simulink model "dut_v7"  (R2023a)
settings: Solver=VariableStepAuto  StartTime=0.0  StopTime=1.0  RelTol=1e-3
undefined symbols (not defined in the file): DiscIntNeverNeededParam, Fs
libraries: hdlsllib x1, simulink_extras x1
settings Model: Creator=pj  LastModifiedBy=maarikazuki
settings ModelReferenceCC: EnableRefExpFcnMdlSchedulingChecks=on

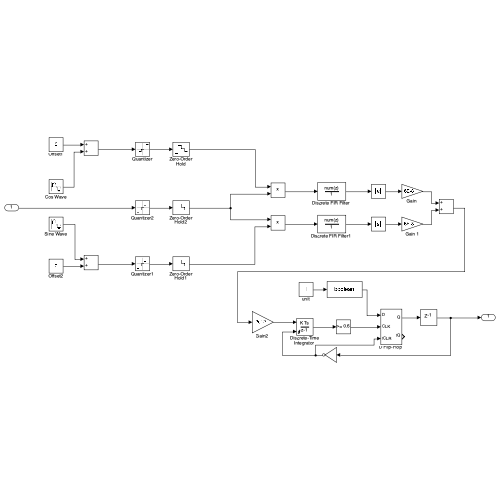
[thumbnail: Simulink's stored preview of the top-level diagram]
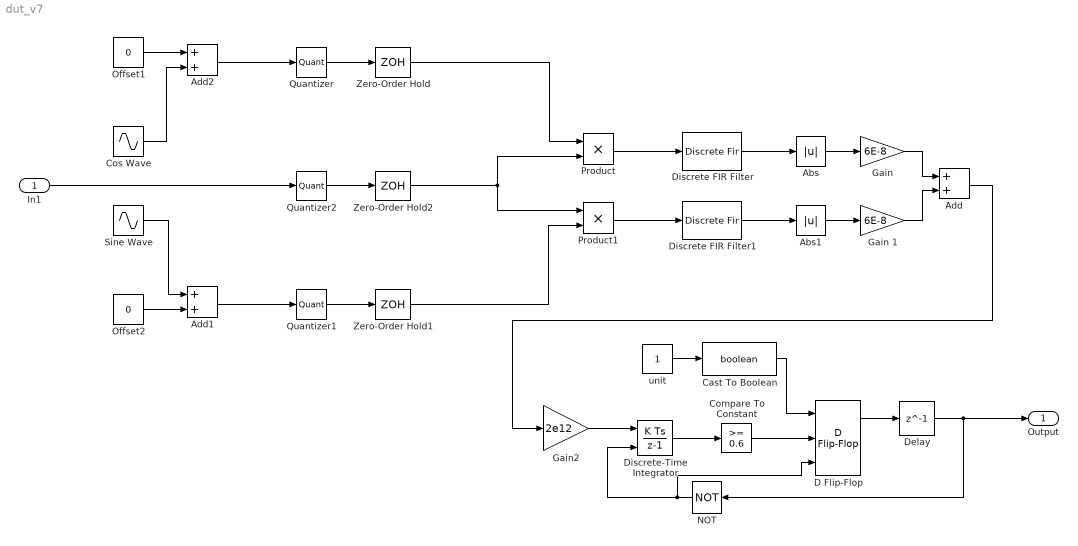
== system dut_v7 ==
  In1 : Inport
  Abs : Abs  SaturateOnIntegerOverflow=off
  Abs1 : Abs  SaturateOnIntegerOverflow=off
  Add : Sum
  Add1 : Sum
  Add2 : Sum
  Cast To Boolean : DataTypeConversion  OutDataTypeStr=boolean  SaturateOnIntegerOverflow=off  RndMeth=Floor
  Compare To Constant : hdlsllib/Logic and Bit Operations/Compare To Constant  relop=>=  const=0.6  OutDataTypeStr=boolean
  Cos Wave : Sin  Frequency=2*pi*500  Phase=pi/2  SampleTime=1/Fs
  "D Flip-Flop " : simulink_extras/Flip Flops/D Flip-Flop
  Delay : Delay  DelayLength=1
  "Discrete FIR Filter " : DiscreteFir  Coefficients="[0.00025758\t1.30E-05\t1.32E-05\t1.36E-05\t1.38E-05\t1.42E-05\t1.45E-05\t1.49E-05\t1.51E-05\t1.56E-05\t1.58E-05\t1.63E-05\t1.66E-05\t1.71E-05\t1.74E-05\t1.79E-05\t1.82E-05\t1.87E-05\t1.88E-05\t1.93E-05\t1.99E-05\t2.02E-05\t2.06E-05\t2.11E-05\t2.15E-05\t2.20E-05\t2.24E-05\t2.29E-05\t2.33E-05\t2.39E-05\t2.42E-05\t2.48E-05\t2.52E-05\t2.57E-05\t2.61E-05\t2.67E-05\t2.72E-05\t2.78E-05\t2.82E-05\t2.88E-05\t2.93E-05\t2.99E-05\t3.03E-05\t3.10E-05\t3.15E-05\t3.21E-05\t3.26E-05\t3.32E-05\t3.37E-05\t3.44E-05\t3.49E-05\t3.56E-05\t3.62E-05\t3.69E-05\t3.74E-05\t3.81E-05\t3.87E-05\t3.94E-05\t4.00E-05\t4.07E-05\t4.13E-05\t4.20E-05\t4.27E-05\t4.34E-05\t4.40E-05\t4.48E-05\t4.55E-05\t4.62E-05\t4.69E-05\t4.77E-05\t4.84E-05\t4.92E-05\t4.99E-05\t5.07E-05\t5.14E-05\t5.22E-05\t5.30E-05\t5.38E-05\t5.45E-05\t5.54E-05\t5.62E-05\t5.71E-05\t5.78E-05\t5.88E-05\t5.95E-05\t6.05E-05\t6.13E-05\t6.22E-05\t6.30E-05\t6.40E-05\t6.48E-05\t6.58E-05\t6.66E-05\t6.76E-05\t6.85E-05\t6.95E-05\t7.04E-05\t7.14E-05\t7.23E-05\t7.34E-05\t7.43E-05\t7.53E-05\t7.63E-05\t7.73E-05\t7.83E-05\t7.94E-05\t8.04E-05\t8.15E-05\t8.25E-05\t8.36E-05\t8.46E-05\t8.57E-05\t8.68E-05\t8.79E-05\t8.90E-05\t9.01E-05\t9.12E-05\t9.24E-05\t9.35E-05\t9.47E-05\t9.58E-05\t9.70E-05\t9.81E-05\t9.94E-05\t0.00010053\t0.00010181\t0.00010296\t0.00010425\t0.00010542\t0.00010673\t0.00010792\t0.00010925\t0.00011046\t0.00011181\t0.00011304\t0.0001144\t0.00011566\t0.00011704\t0.00011832\t0.00011972\t0.00012101\t0.00012243\t0.00012374\t0.00012519\t0.00012652\t0.00012798\t0.00012933\t0.00013081\t0.00013218\t0.00013368\t0.00013507\t0.00013659\t0.000138\t0.00013954\t0.00014097\t0.00014253\t0.00014398\t0.00014556\t0.00014703\t0.00014863\t0.00015012\t0.00015173\t0.00015325\t0.00015488\t0.00015642\t0.00015807\t0.00015963\t0.0001613\t0.00016288\t0.00016457\t0.00016617\t0.00016788\t0.0001695\t0.00017123\t0.00017287\t0.00017462\t0.00017628\t0.00017805\t0.00017974\t0.00018153\t0.00018323\t0.00018504\t0.00018676\t0.00018859\t0.00019034\t0.00019218\t0.00019395\t0.00019582\t0.00019761\t0.00019949\t0.0002013\t0.00020321\t0.00020504\t0.00020697\t0.00020882\t0.00021077\t0.00021264\t0.00021461\t0.0002165\t0.00021849\t0.0002204\t0.00022241\t0.00022434\t0.00022637\t0.00022832\t0.00023037\t0.00023235\t0.00023441\t0.00023641\t0.00023849\t0.00024051\t0.00024261\t0.00024465\t0.00024678\t0.00024883\t0.00025098\t0.00025306\t0.00025522\t0.00025732\t0.0002595\t0.00026162\t0.00026382\t0.00026596\t0.00026818\t0.00027034\t0.00027258\t0.00027476\t0.00027701\t0.00027921\t0.00028149\t0.00028371\t0.000286\t0.00028824\t0.00029056\t0.00029282\t0.00029515\t0.00029743\t0.00029978\t0.00030207\t0.00030444\t0.00030676\t0.00030915\t0.00031148\t0.00031389\t0.00031624\t0.00031866\t0.00032104\t0.00032348\t0.00032587\t0.00032833\t0.00033074\t0.00033322\t0.00033565\t0.00033814\t0.00034059\t0.0003431\t0.00034556\t0.00034809\t0.00035058\t0.00035312\t0.00035562\t0.00035819\t0.00036071\t0.00036328\t0.00036582\t0.00036842\t0.00037097\t0.00037358\t0.00037615\t0.00037878\t0.00038137\t0.00038401\t0.00038662\t0.00038927\t0.00039189\t0.00039457\t0.00039721\t0.0003999\t0.00040255\t0.00040525\t0.00040792\t0.00041064\t0.00041333\t0.00041606\t0.00041876\t0.00042151\t0.00042422\t0.00042699\t0.00042972\t0.00043249\t0.00043524\t0.00043803\t0.00044079\t0.00044359\t0.00044636\t0.00044918\t0.00045197\t0.0004548\t0.0004576\t0.00046044\t0.00046325\t0.00046611\t0.00046894\t0.0004718\t0.00047464\t0.00047752\t0.00048037\t0.00048327\t0.00048613\t0.00048903\t0.00049191\t0.00049482\t0.00049771\t0.00050063\t0.00050353\t0.00050647\t0.00050938\t0.00051232\t0.00051524\t0.0005182\t0.00052113\t0.0005241\t0.00052703\t0.00053001\t0.00053296\t0.00053595\t0.0005389\t0.0005419\t0.00054486\t0.00054787\t0.00055084\t0.00055386\t0.00055684\t0.00055986\t0.00056285\t0.00056588\t0.00056888\t0.00057191\t0.00057492\t0.00057796\t0.00058097\t0.00058402\t0.00058704\t0.0005901\t0.00059312\t0.00059618\t0.00059922\t0.00060228\t0.00060532\t0.00060839\t0.00061144\t0.00061451\t0.00061756\t0.00062064\t0.00062369\t0.00062678\t0.00062984\t0.00063293\t0.00063599\t0.00063908\t0.00064214\t0.00064524\t0.00064831\t0.0006514\t0.00065447\t0.00065757\t0.00066065\t0.00066375\t0.00066682\t0.00066993\t0.000673\t0.00067611\t0.00067919\t0.00068229\t0.00068537\t0.00068847\t0.00069155\t0.00069466\t0.00069774\t0.00070084\t0.00070392\t0.00070702\t0.0007101\t0.0007132\t0.00071628\t0.00071938\t0.00072245\t0.00072555\t0.00072862\t0.00073172\t0.00073479\t0.00073788\t0.00074094\t0.00074404\t0.0007471\t0.00075018\t0.00075324\t0.00075632\t0.00075938\t0.00076246\t0.0007655\t0.00076858\t0.00077162\t0.00077469\t0.00077773\t0.00078079\t0.00078382\t0.00078688\t0.0007899\t0.00079295\t0.00079597\t0.00079902\t0.00080203\t0.00080506\t0.00080807\t0.00081109\t0.00081409\t0.00081711\t0.00082009\t0.00082311\t0.00082608\t0.00082909\t0.00083205\t0.00083505\t0.000838\t0.00084099\t0.00084394\t0.00084691\t0.00084985\t0.00085281\t0.00085573\t0.00085868\t0.0008616\t0.00086454\t0.00086744\t0.00087037\t0.00087326\t0.00087617\t0.00087905\t0.00088195\t0.00088481\t0.0008877\t0.00089055\t0.00089342\t0.00089626\t0.00089912\t0.00090194\t0.00090479\t0.00090759\t0.00091042\t0.00091321\t0.00091603\t0.0009188\t0.0009216\t0.00092436\t0.00092714\t0.00092989\t0.00093265\t0.00093538\t0.00093812\t0.00094083\t0.00094356\t0.00094625\t0.00094896\t0.00095164\t0.00095433\t0.00095698\t0.00095966\t0.00096229\t0.00096495\t0.00096756\t0.0009702\t0.00097279\t0.0009754\t0.00097798\t0.00098057\t0.00098313\t0.0009857\t0.00098823\t0.00099079\t0.0009933\t0.00099583\t0.00099832\t0.0010008\t0.0010033\t0.0010058\t0.0010082\t0.0010107\t0.0010131\t0.0010155\t0.0010179\t0.0010204\t0.0010227\t0.0010251\t0.0010275\t0.0010298\t0.0010322\t0.0010345\t0.0010368\t0.0010391\t0.0010414\t0.0010437\t0.0010459\t0.0010482\t0.0010504\t0.0010527\t0.0010549\t0.0010571\t0.0010592\t0.0010614\t0.0010636\t0.0010657\t0.0010678\t0.00107\t0.0010721\t0.0010742\t0.0010762\t0.0010783\t0.0010803\t0.0010824\t0.0010844\t0.0010864\t0.0010883\t0.0010903\t0.0010923\t0.0010942\t0.0010961\t0.0010981\t0.0011\t0.0011018\t0.0011037\t0.0011056\t0.0011074\t0.0011092\t0.001111\t0.0011128\t0.0011146\t0.0011163\t0.0011181\t0.0011198\t0.0011215\t0.0011232\t0.0011249\t0.0011265\t0.0011282\t0.0011298\t0.0011314\t0.001133\t0.0011346\t0.0011362\t0.0011377\t0.0011392\t0.0011407\t0.0011422\t0.0011437\t0.0011452\t0.0011466\t0.001148\t0.0011494\t0.0011508\t0.0011522\t0.0011536\t0.0011549\t0.0011562\t0.0011575\t0.0011588\t0.0011601\t0.0011613\t0.0011626\t0.0011638\t0.001165\t0.0011662\t0.0011673\t0.0011685\t0.0011696\t0.0011707\t0.0011718\t0.0011729\t0.0011739\t0.0011749\t0.0011759\t0.0011769\t0.0011779\t0.0011789\t0.0011798\t0.0011808\t0.0011816\t0.0011825\t0.0011834\t0.0011843\t0.0011851\t0.0011859\t0.0011867\t0.0011875\t0.0011882\t0.0011889\t0.0011897\t0.0011904\t0.001191\t0.0011917\t0.0011923\t0.001193\t0.0011936\t0.0011941\t0.0011947\t0.0011953\t0.0011958\t0.0011963\t0.0011968\t0.0011972\t0.0011977\t0.0011981\t0.0011985\t0.0011989\t0.0011993\t0.0011996\t0.0012\t0.0012003\t0.0012006\t0.0012008\t0.0012011\t0.0012013\t0.0012015\t0.0012017\t0.0012019\t0.0012021\t0.0012022\t0.0012023\t0.0012024\t0.0012025\t0.0012026\t0.0012026\t0.0012026\t0.0012026\t0.0012026\t0.0012026\t0.0012025\t0.0012024\t0.0012023\t0.0012022\t0.0012021\t0.0012019\t0.0012017\t0.0012015\t0.0012013\t0.0012011\t0.0012008\t0.0012006\t0.0012003\t0.0012\t0.0011996\t0.0011993\t0.0011989\t0.0011985\t0.0011981\t0.0011977\t0.0011972\t0.0011968\t0.0011963\t0.0011958\t0.0011953\t0.0011947\t0.0011941\t0.0011936\t0.001193\t0.0011923\t0.0011917\t0.001191\t0.0011904\t0.0011897\t0.0011889\t0.0011882\t0.0011875\t0.0011867\t0.0011859\t0.0011851\t0.0011843\t0.0011834\t0.0011825\t0.0011816\t0.0011808\t0.0011798\t0.0011789\t0.0011779\t0.0011769\t0.0011759\t0.0011749\t0.0011739\t0.0011729\t0.0011718\t0.0011707\t0.0011696\t0.0011685\t0.0011673\t0.0011662\t0.001165\t0.0011638\t0.0011626\t0.0011613\t0.0011601\t0.0011588\t0.0011575\t0.0011562\t0.0011549\t0.0011536\t0.0011522\t0.0011508\t0.0011494\t0.001148\t0.0011466\t0.0011452\t0.0011437\t0.0011422\t0.0011407\t0.0011392\t0.0011377\t0.0011362\t0.0011346\t0.001133\t0.0011314\t0.0011298\t0.0011282\t0.0011265\t0.0011249\t0.0011232\t0.0011215\t0.0011198\t0.0011181\t0.0011163\t0.0011146\t0.0011128\t0.001111\t0.0011092\t0.0011074\t0.0011056\t0.0011037\t0.0011018\t0.0011\t0.0010981\t0.0010961\t0.0010942\t0.0010923\t0.0010903\t0.0010883\t0.0010864\t0.0010844\t0.0010824\t0.0010803\t0.0010783\t0.0010762\t0.0010742\t0.0010721\t0.00107\t0.0010678\t0.0010657\t0.0010636\t0.0010614\t0.0010592\t0.0010571\t0.0010549\t0.0010527\t0.0010504\t0.0010482\t0.0010459\t0.0010437\t0.0010414\t0.0010391\t0.0010368\t0.0010345\t0.0010322\t0.0010298\t0.0010275\t0.0010251\t0.0010227\t0.0010204\t0.0010179\t0.0010155\t0.0010131\t0.0010107\t0.0010082\t0.0010058\t0.0010033\t0.0010008\t0.00099832\t0.00099583\t0.0009933\t0.00099079\t0.00098823\t0.0009857\t0.00098313\t0.00098057\t0.00097798\t0.0009754\t0.00097279\t0.0009702\t0.00096756\t0.00096495\t0.00096229\t0.00095966\t0.00095698\t0.00095433\t0.00095164\t0.00094896\t0.00094625\t0.00094356\t0.00094083\t0.00093812\t0.00093538\t0.00093265\t0.00092989\t0.00092714\t0.00092436\t0.0009216\t0.0009188\t0.00091603\t0.00091321\t0.00091042\t0.00090759\t0.00090479\t0.00090194\t0.00089912\t0.00089626\t0.00089342\t0.00089055\t0.0008877\t0.00088481\t0.00088195\t0.00087905\t0.00087617\t0.00087326\t0.00087037\t0.00086744\t0.00086454\t0.0008616\t0.00085868\t0.00085573\t0.00085281\t0.00084985\t0.00084691\t0.00084394\t0.00084099\t0.000838\t0.00083505\t0.00083205\t0.00082909\t0.00082608\t0.00082311\t0.00082009\t0.00081711\t0.00081409\t0.00081109\t0.00080807\t0.00080506\t0.00080203\t0.00079902\t0.00079597\t0.00079295\t0.0007899\t0.00078688\t0.00078382\t0.00078079\t0.00077773\t0.00077469\t0.00077162\t0.00076858\t0.0007655\t0.00076246\t0.00075938\t0.00075632\t0.00075324\t0.00075018\t0.0007471\t0.00074404\t0.00074094\t0.00073788\t0.00073479\t0.00073172\t0.00072862\t0.00072555\t0.00072245\t0.00071938\t0.00071628\t0.0007132\t0.0007101\t0.00070702\t0.00070392\t0.00070084\t0.00069774\t0.00069466\t0.00069155\t0.00068847\t0.00068537\t0.00068229\t0.00067919\t0.00067611\t0.000673\t0.00066993\t0.00066682\t0.00066375\t0.00066065\t0.00065757\t0.00065447\t0.0006514\t0.00064831\t0.00064524\t0.00064214\t0.00063908\t0.00063599\t0.00063293\t0.00062984\t0.00062678\t0.00062369\t0.00062064\t0.00061756\t0.00061451\t0.00061144\t0.00060839\t0.00060532\t0.00060228\t0.00059922\t0.00059618\t0.00059312\t0.0005901\t0.00058704\t0.00058402\t0.00058097\t0.00057796\t0.00057492\t0.00057191\t0.00056888\t0.00056588\t0.00056285\t0.00055986\t0.00055684\t0.00055386\t0.00055084\t0.00054787\t0.00054486\t0.0005419\t0.0005389\t0.00053595\t0.00053296\t0.00053001\t0.00052703\t0.0005241\t0.00052113\t0.0005182\t0.00051524\t0.00051232\t0.00050938\t0.00050647\t0.00050353\t0.00050063\t0.00049771\t0.00049482\t0.00049191\t0.00048903\t0.00048613\t0.00048327\t0.00048037\t0.00047752\t0.00047464\t0.0004718\t0.00046894\t0.00046611\t0.00046325\t0.00046044\t0.0004576\t0.0004548\t0.00045197\t0.00044918\t0.00044636\t0.00044359\t0.00044079\t0.00043803\t0.00043524\t0.00043249\t0.00042972\t0.00042699\t0.00042422\t0.00042151\t0.00041876\t0.00041606\t0.00041333\t0.00041064\t0.00040792\t0.00040525\t0.00040255\t0.0003999\t0.00039721\t0.00039457\t0.00039189\t0.00038927\t0.00038662\t0.00038401\t0.00038137\t0.00037878\t0.00037615\t0.00037358\t0.00037097\t0.00036842\t0.00036582\t0.00036328\t0.00036071\t0.00035819\t0.00035562\t0.00035312\t0.00035058\t0.00034809\t0.00034556\t0.0003431\t0.00034059\t0.00033814\t0.00033565\t0.00033322\t0.00033074\t0.00032833\t0.00032587\t0.00032348\t0.00032104\t0.00031866\t0.00031624\t0.00031389\t0.00031148\t0.00030915\t0.00030676\t0.00030444\t0.00030207\t0.00029978\t0.00029743\t0.00029515\t0.00029282\t0.00029056\t0.00028824\t0.000286\t0.00028371\t0.00028149\t0.00027921\t0.00027701\t0.00027476\t0.00027258\t0.00027034\t0.00026818\t0.00026596\t0.00026382\t0.00026162\t0.0002595\t0.00025732\t0.00025522\t0.00025306\t0.00025098\t0.00024883\t0.00024678\t0.00024465\t0.00024261\t0.00024051\t0.00023849\t0.00023641\t0.00023441\t0.00023235\t0.00023037\t0.00022832\t0.00022637\t0.00022434\t0.00022241\t0.0002204\t0.00021849\t0.0002165\t0.00021461\t0.00021264\t0.00021077\t0.00020882\t0.00020697\t0.00020504\t0.00020321\t0.0002013\t0.00019949\t0.00019761\t0.00019582\t0.00019395\t0.00019218\t0.00019034\t0.00018859\t0.00018676\t0.00018504\t0.00018323\t0.00018153\t0.00017974\t0.00017805\t0.00017628\t0.00017462\t0.00017287\t0.00017123\t0.0001695\t0.00016788\t0.00016617\t0.00016457\t0.00016288\t0.0001613\t0.00015963\t0.00015807\t0.00015642\t0.00015488\t0.00015325\t0.00015173\t0.00015012\t0.00014863\t0.00014703\t0.00014556\t0.00014398\t0.00014253\t0.00014097\t0.00013954\t0.000138\t0.00013659\t0.00013507\t0.00013368\t0.00013218\t0.00013081\t0.00012933\t0.00012798\t0.00012652\t0.00012519\t0.00012374\t0.00012243\t0.00012101\t0.00011972\t0.00011832\t0.00011704\t0.00011566\t0.0001144\t0.00011304\t0.00011181\t0.00011046\t0.00010925\t0.00010792\t0.00010673\t0.00010542\t0.00010425\t0.00010296\t0.00010181\t0.00010053\t9.94E-05\t9.81E-05\t9.70E-05\t9.58E-05\t9.47E-05\t9.35E-05\t9.24E-05\t9.12E-05\t9.01E-05\t8.90E-05\t8.79E-05\t8.68E-05\t8.57E-05\t8.46E-05\t8.36E-05\t8.25E-05\t8.15E-05\t8.04E-05\t7.94E-05\t7.83E-05\t7.73E-05\t7.63E-05\t7.53E-05\t7.43E-05\t7.34E-05\t7.23E-05\t7.14E-05\t7.04E-05\t6.95E-05\t6.85E-05\t6.76E-05\t6.66E-05\t6.58E-05\t6.48E-05\t6.40E-05\t6.30E-05\t6.22E-05\t6.13E-05\t6.05E-05\t5.95E-05\t5.88E-05\t5.78E-05\t5.71E-05\t5.62E-05\t5.54E-05\t5.45E-05\t5.38E-05\t5.30E-05\t5.22E-05\t5.14E-05\t5.07E-05\t4.99E-05\t4.92E-05\t4.84E-05\t4.77E-05\t4.69E-05\t4.62E-05\t4.55E-05\t4.48E-05\t4.40E-05\t4.34E-05\t4.27E-05\t4.20E-05\t4.13E-05\t4.07E-05\t4.00E-05\t3.94E-05\t3.87E-05\t3.81E-05\t3.74E-05\t3.69E-05\t3.62E-05\t3.56E-05\t3.49E-05\t3.44E-05\t3.37E-05\t3.32E-05\t3.26E-05\t3.21E-05\t3.15E-05\t3.10E-05\t3.03E-05\t2.99E-05\t2.93E-05\t2.88E-05\t2.82E-05\t2.78E-05\t2.72E-05\t2.67E-05\t2.61E-05\t2.57E-05\t2.52E-05\t2.48E-05\t2.42E-05\t2.39E-05\t2.33E-05\t2.29E-05\t2.24E-05\t2.20E-05\t2.15E-05\t2.11E-05\t2.06E-05\t2.02E-05\t1.99E-05\t1.93E-05\t1.88E-05\t1.87E-05\t1.82E-05\t1.79E-05\t1.74E-05\t1.71E-05\t1.66E-05\t1.63E-05\t1.58E-05\t1.56E-05\t1.51E-05\t1.49E-05\t1.45E-05\t1.42E-05\t1.38E-05\t1.36E-05\t1.32E-05\t1.30E-05\t0.00025758]"
  "Discrete FIR Filter1 " : DiscreteFir  Coefficients="[0.00025758\t1.30E-05\t1.32E-05\t1.36E-05\t1.38E-05\t1.42E-05\t1.45E-05\t1.49E-05\t1.51E-05\t1.56E-05\t1.58E-05\t1.63E-05\t1.66E-05\t1.71E-05\t1.74E-05\t1.79E-05\t1.82E-05\t1.87E-05\t1.88E-05\t1.93E-05\t1.99E-05\t2.02E-05\t2.06E-05\t2.11E-05\t2.15E-05\t2.20E-05\t2.24E-05\t2.29E-05\t2.33E-05\t2.39E-05\t2.42E-05\t2.48E-05\t2.52E-05\t2.57E-05\t2.61E-05\t2.67E-05\t2.72E-05\t2.78E-05\t2.82E-05\t2.88E-05\t2.93E-05\t2.99E-05\t3.03E-05\t3.10E-05\t3.15E-05\t3.21E-05\t3.26E-05\t3.32E-05\t3.37E-05\t3.44E-05\t3.49E-05\t3.56E-05\t3.62E-05\t3.69E-05\t3.74E-05\t3.81E-05\t3.87E-05\t3.94E-05\t4.00E-05\t4.07E-05\t4.13E-05\t4.20E-05\t4.27E-05\t4.34E-05\t4.40E-05\t4.48E-05\t4.55E-05\t4.62E-05\t4.69E-05\t4.77E-05\t4.84E-05\t4.92E-05\t4.99E-05\t5.07E-05\t5.14E-05\t5.22E-05\t5.30E-05\t5.38E-05\t5.45E-05\t5.54E-05\t5.62E-05\t5.71E-05\t5.78E-05\t5.88E-05\t5.95E-05\t6.05E-05\t6.13E-05\t6.22E-05\t6.30E-05\t6.40E-05\t6.48E-05\t6.58E-05\t6.66E-05\t6.76E-05\t6.85E-05\t6.95E-05\t7.04E-05\t7.14E-05\t7.23E-05\t7.34E-05\t7.43E-05\t7.53E-05\t7.63E-05\t7.73E-05\t7.83E-05\t7.94E-05\t8.04E-05\t8.15E-05\t8.25E-05\t8.36E-05\t8.46E-05\t8.57E-05\t8.68E-05\t8.79E-05\t8.90E-05\t9.01E-05\t9.12E-05\t9.24E-05\t9.35E-05\t9.47E-05\t9.58E-05\t9.70E-05\t9.81E-05\t9.94E-05\t0.00010053\t0.00010181\t0.00010296\t0.00010425\t0.00010542\t0.00010673\t0.00010792\t0.00010925\t0.00011046\t0.00011181\t0.00011304\t0.0001144\t0.00011566\t0.00011704\t0.00011832\t0.00011972\t0.00012101\t0.00012243\t0.00012374\t0.00012519\t0.00012652\t0.00012798\t0.00012933\t0.00013081\t0.00013218\t0.00013368\t0.00013507\t0.00013659\t0.000138\t0.00013954\t0.00014097\t0.00014253\t0.00014398\t0.00014556\t0.00014703\t0.00014863\t0.00015012\t0.00015173\t0.00015325\t0.00015488\t0.00015642\t0.00015807\t0.00015963\t0.0001613\t0.00016288\t0.00016457\t0.00016617\t0.00016788\t0.0001695\t0.00017123\t0.00017287\t0.00017462\t0.00017628\t0.00017805\t0.00017974\t0.00018153\t0.00018323\t0.00018504\t0.00018676\t0.00018859\t0.00019034\t0.00019218\t0.00019395\t0.00019582\t0.00019761\t0.00019949\t0.0002013\t0.00020321\t0.00020504\t0.00020697\t0.00020882\t0.00021077\t0.00021264\t0.00021461\t0.0002165\t0.00021849\t0.0002204\t0.00022241\t0.00022434\t0.00022637\t0.00022832\t0.00023037\t0.00023235\t0.00023441\t0.00023641\t0.00023849\t0.00024051\t0.00024261\t0.00024465\t0.00024678\t0.00024883\t0.00025098\t0.00025306\t0.00025522\t0.00025732\t0.0002595\t0.00026162\t0.00026382\t0.00026596\t0.00026818\t0.00027034\t0.00027258\t0.00027476\t0.00027701\t0.00027921\t0.00028149\t0.00028371\t0.000286\t0.00028824\t0.00029056\t0.00029282\t0.00029515\t0.00029743\t0.00029978\t0.00030207\t0.00030444\t0.00030676\t0.00030915\t0.00031148\t0.00031389\t0.00031624\t0.00031866\t0.00032104\t0.00032348\t0.00032587\t0.00032833\t0.00033074\t0.00033322\t0.00033565\t0.00033814\t0.00034059\t0.0003431\t0.00034556\t0.00034809\t0.00035058\t0.00035312\t0.00035562\t0.00035819\t0.00036071\t0.00036328\t0.00036582\t0.00036842\t0.00037097\t0.00037358\t0.00037615\t0.00037878\t0.00038137\t0.00038401\t0.00038662\t0.00038927\t0.00039189\t0.00039457\t0.00039721\t0.0003999\t0.00040255\t0.00040525\t0.00040792\t0.00041064\t0.00041333\t0.00041606\t0.00041876\t0.00042151\t0.00042422\t0.00042699\t0.00042972\t0.00043249\t0.00043524\t0.00043803\t0.00044079\t0.00044359\t0.00044636\t0.00044918\t0.00045197\t0.0004548\t0.0004576\t0.00046044\t0.00046325\t0.00046611\t0.00046894\t0.0004718\t0.00047464\t0.00047752\t0.00048037\t0.00048327\t0.00048613\t0.00048903\t0.00049191\t0.00049482\t0.00049771\t0.00050063\t0.00050353\t0.00050647\t0.00050938\t0.00051232\t0.00051524\t0.0005182\t0.00052113\t0.0005241\t0.00052703\t0.00053001\t0.00053296\t0.00053595\t0.0005389\t0.0005419\t0.00054486\t0.00054787\t0.00055084\t0.00055386\t0.00055684\t0.00055986\t0.00056285\t0.00056588\t0.00056888\t0.00057191\t0.00057492\t0.00057796\t0.00058097\t0.00058402\t0.00058704\t0.0005901\t0.00059312\t0.00059618\t0.00059922\t0.00060228\t0.00060532\t0.00060839\t0.00061144\t0.00061451\t0.00061756\t0.00062064\t0.00062369\t0.00062678\t0.00062984\t0.00063293\t0.00063599\t0.00063908\t0.00064214\t0.00064524\t0.00064831\t0.0006514\t0.00065447\t0.00065757\t0.00066065\t0.00066375\t0.00066682\t0.00066993\t0.000673\t0.00067611\t0.00067919\t0.00068229\t0.00068537\t0.00068847\t0.00069155\t0.00069466\t0.00069774\t0.00070084\t0.00070392\t0.00070702\t0.0007101\t0.0007132\t0.00071628\t0.00071938\t0.00072245\t0.00072555\t0.00072862\t0.00073172\t0.00073479\t0.00073788\t0.00074094\t0.00074404\t0.0007471\t0.00075018\t0.00075324\t0.00075632\t0.00075938\t0.00076246\t0.0007655\t0.00076858\t0.00077162\t0.00077469\t0.00077773\t0.00078079\t0.00078382\t0.00078688\t0.0007899\t0.00079295\t0.00079597\t0.00079902\t0.00080203\t0.00080506\t0.00080807\t0.00081109\t0.00081409\t0.00081711\t0.00082009\t0.00082311\t0.00082608\t0.00082909\t0.00083205\t0.00083505\t0.000838\t0.00084099\t0.00084394\t0.00084691\t0.00084985\t0.00085281\t0.00085573\t0.00085868\t0.0008616\t0.00086454\t0.00086744\t0.00087037\t0.00087326\t0.00087617\t0.00087905\t0.00088195\t0.00088481\t0.0008877\t0.00089055\t0.00089342\t0.00089626\t0.00089912\t0.00090194\t0.00090479\t0.00090759\t0.00091042\t0.00091321\t0.00091603\t0.0009188\t0.0009216\t0.00092436\t0.00092714\t0.00092989\t0.00093265\t0.00093538\t0.00093812\t0.00094083\t0.00094356\t0.00094625\t0.00094896\t0.00095164\t0.00095433\t0.00095698\t0.00095966\t0.00096229\t0.00096495\t0.00096756\t0.0009702\t0.00097279\t0.0009754\t0.00097798\t0.00098057\t0.00098313\t0.0009857\t0.00098823\t0.00099079\t0.0009933\t0.00099583\t0.00099832\t0.0010008\t0.0010033\t0.0010058\t0.0010082\t0.0010107\t0.0010131\t0.0010155\t0.0010179\t0.0010204\t0.0010227\t0.0010251\t0.0010275\t0.0010298\t0.0010322\t0.0010345\t0.0010368\t0.0010391\t0.0010414\t0.0010437\t0.0010459\t0.0010482\t0.0010504\t0.0010527\t0.0010549\t0.0010571\t0.0010592\t0.0010614\t0.0010636\t0.0010657\t0.0010678\t0.00107\t0.0010721\t0.0010742\t0.0010762\t0.0010783\t0.0010803\t0.0010824\t0.0010844\t0.0010864\t0.0010883\t0.0010903\t0.0010923\t0.0010942\t0.0010961\t0.0010981\t0.0011\t0.0011018\t0.0011037\t0.0011056\t0.0011074\t0.0011092\t0.001111\t0.0011128\t0.0011146\t0.0011163\t0.0011181\t0.0011198\t0.0011215\t0.0011232\t0.0011249\t0.0011265\t0.0011282\t0.0011298\t0.0011314\t0.001133\t0.0011346\t0.0011362\t0.0011377\t0.0011392\t0.0011407\t0.0011422\t0.0011437\t0.0011452\t0.0011466\t0.001148\t0.0011494\t0.0011508\t0.0011522\t0.0011536\t0.0011549\t0.0011562\t0.0011575\t0.0011588\t0.0011601\t0.0011613\t0.0011626\t0.0011638\t0.001165\t0.0011662\t0.0011673\t0.0011685\t0.0011696\t0.0011707\t0.0011718\t0.0011729\t0.0011739\t0.0011749\t0.0011759\t0.0011769\t0.0011779\t0.0011789\t0.0011798\t0.0011808\t0.0011816\t0.0011825\t0.0011834\t0.0011843\t0.0011851\t0.0011859\t0.0011867\t0.0011875\t0.0011882\t0.0011889\t0.0011897\t0.0011904\t0.001191\t0.0011917\t0.0011923\t0.001193\t0.0011936\t0.0011941\t0.0011947\t0.0011953\t0.0011958\t0.0011963\t0.0011968\t0.0011972\t0.0011977\t0.0011981\t0.0011985\t0.0011989\t0.0011993\t0.0011996\t0.0012\t0.0012003\t0.0012006\t0.0012008\t0.0012011\t0.0012013\t0.0012015\t0.0012017\t0.0012019\t0.0012021\t0.0012022\t0.0012023\t0.0012024\t0.0012025\t0.0012026\t0.0012026\t0.0012026\t0.0012026\t0.0012026\t0.0012026\t0.0012025\t0.0012024\t0.0012023\t0.0012022\t0.0012021\t0.0012019\t0.0012017\t0.0012015\t0.0012013\t0.0012011\t0.0012008\t0.0012006\t0.0012003\t0.0012\t0.0011996\t0.0011993\t0.0011989\t0.0011985\t0.0011981\t0.0011977\t0.0011972\t0.0011968\t0.0011963\t0.0011958\t0.0011953\t0.0011947\t0.0011941\t0.0011936\t0.001193\t0.0011923\t0.0011917\t0.001191\t0.0011904\t0.0011897\t0.0011889\t0.0011882\t0.0011875\t0.0011867\t0.0011859\t0.0011851\t0.0011843\t0.0011834\t0.0011825\t0.0011816\t0.0011808\t0.0011798\t0.0011789\t0.0011779\t0.0011769\t0.0011759\t0.0011749\t0.0011739\t0.0011729\t0.0011718\t0.0011707\t0.0011696\t0.0011685\t0.0011673\t0.0011662\t0.001165\t0.0011638\t0.0011626\t0.0011613\t0.0011601\t0.0011588\t0.0011575\t0.0011562\t0.0011549\t0.0011536\t0.0011522\t0.0011508\t0.0011494\t0.001148\t0.0011466\t0.0011452\t0.0011437\t0.0011422\t0.0011407\t0.0011392\t0.0011377\t0.0011362\t0.0011346\t0.001133\t0.0011314\t0.0011298\t0.0011282\t0.0011265\t0.0011249\t0.0011232\t0.0011215\t0.0011198\t0.0011181\t0.0011163\t0.0011146\t0.0011128\t0.001111\t0.0011092\t0.0011074\t0.0011056\t0.0011037\t0.0011018\t0.0011\t0.0010981\t0.0010961\t0.0010942\t0.0010923\t0.0010903\t0.0010883\t0.0010864\t0.0010844\t0.0010824\t0.0010803\t0.0010783\t0.0010762\t0.0010742\t0.0010721\t0.00107\t0.0010678\t0.0010657\t0.0010636\t0.0010614\t0.0010592\t0.0010571\t0.0010549\t0.0010527\t0.0010504\t0.0010482\t0.0010459\t0.0010437\t0.0010414\t0.0010391\t0.0010368\t0.0010345\t0.0010322\t0.0010298\t0.0010275\t0.0010251\t0.0010227\t0.0010204\t0.0010179\t0.0010155\t0.0010131\t0.0010107\t0.0010082\t0.0010058\t0.0010033\t0.0010008\t0.00099832\t0.00099583\t0.0009933\t0.00099079\t0.00098823\t0.0009857\t0.00098313\t0.00098057\t0.00097798\t0.0009754\t0.00097279\t0.0009702\t0.00096756\t0.00096495\t0.00096229\t0.00095966\t0.00095698\t0.00095433\t0.00095164\t0.00094896\t0.00094625\t0.00094356\t0.00094083\t0.00093812\t0.00093538\t0.00093265\t0.00092989\t0.00092714\t0.00092436\t0.0009216\t0.0009188\t0.00091603\t0.00091321\t0.00091042\t0.00090759\t0.00090479\t0.00090194\t0.00089912\t0.00089626\t0.00089342\t0.00089055\t0.0008877\t0.00088481\t0.00088195\t0.00087905\t0.00087617\t0.00087326\t0.00087037\t0.00086744\t0.00086454\t0.0008616\t0.00085868\t0.00085573\t0.00085281\t0.00084985\t0.00084691\t0.00084394\t0.00084099\t0.000838\t0.00083505\t0.00083205\t0.00082909\t0.00082608\t0.00082311\t0.00082009\t0.00081711\t0.00081409\t0.00081109\t0.00080807\t0.00080506\t0.00080203\t0.00079902\t0.00079597\t0.00079295\t0.0007899\t0.00078688\t0.00078382\t0.00078079\t0.00077773\t0.00077469\t0.00077162\t0.00076858\t0.0007655\t0.00076246\t0.00075938\t0.00075632\t0.00075324\t0.00075018\t0.0007471\t0.00074404\t0.00074094\t0.00073788\t0.00073479\t0.00073172\t0.00072862\t0.00072555\t0.00072245\t0.00071938\t0.00071628\t0.0007132\t0.0007101\t0.00070702\t0.00070392\t0.00070084\t0.00069774\t0.00069466\t0.00069155\t0.00068847\t0.00068537\t0.00068229\t0.00067919\t0.00067611\t0.000673\t0.00066993\t0.00066682\t0.00066375\t0.00066065\t0.00065757\t0.00065447\t0.0006514\t0.00064831\t0.00064524\t0.00064214\t0.00063908\t0.00063599\t0.00063293\t0.00062984\t0.00062678\t0.00062369\t0.00062064\t0.00061756\t0.00061451\t0.00061144\t0.00060839\t0.00060532\t0.00060228\t0.00059922\t0.00059618\t0.00059312\t0.0005901\t0.00058704\t0.00058402\t0.00058097\t0.00057796\t0.00057492\t0.00057191\t0.00056888\t0.00056588\t0.00056285\t0.00055986\t0.00055684\t0.00055386\t0.00055084\t0.00054787\t0.00054486\t0.0005419\t0.0005389\t0.00053595\t0.00053296\t0.00053001\t0.00052703\t0.0005241\t0.00052113\t0.0005182\t0.00051524\t0.00051232\t0.00050938\t0.00050647\t0.00050353\t0.00050063\t0.00049771\t0.00049482\t0.00049191\t0.00048903\t0.00048613\t0.00048327\t0.00048037\t0.00047752\t0.00047464\t0.0004718\t0.00046894\t0.00046611\t0.00046325\t0.00046044\t0.0004576\t0.0004548\t0.00045197\t0.00044918\t0.00044636\t0.00044359\t0.00044079\t0.00043803\t0.00043524\t0.00043249\t0.00042972\t0.00042699\t0.00042422\t0.00042151\t0.00041876\t0.00041606\t0.00041333\t0.00041064\t0.00040792\t0.00040525\t0.00040255\t0.0003999\t0.00039721\t0.00039457\t0.00039189\t0.00038927\t0.00038662\t0.00038401\t0.00038137\t0.00037878\t0.00037615\t0.00037358\t0.00037097\t0.00036842\t0.00036582\t0.00036328\t0.00036071\t0.00035819\t0.00035562\t0.00035312\t0.00035058\t0.00034809\t0.00034556\t0.0003431\t0.00034059\t0.00033814\t0.00033565\t0.00033322\t0.00033074\t0.00032833\t0.00032587\t0.00032348\t0.00032104\t0.00031866\t0.00031624\t0.00031389\t0.00031148\t0.00030915\t0.00030676\t0.00030444\t0.00030207\t0.00029978\t0.00029743\t0.00029515\t0.00029282\t0.00029056\t0.00028824\t0.000286\t0.00028371\t0.00028149\t0.00027921\t0.00027701\t0.00027476\t0.00027258\t0.00027034\t0.00026818\t0.00026596\t0.00026382\t0.00026162\t0.0002595\t0.00025732\t0.00025522\t0.00025306\t0.00025098\t0.00024883\t0.00024678\t0.00024465\t0.00024261\t0.00024051\t0.00023849\t0.00023641\t0.00023441\t0.00023235\t0.00023037\t0.00022832\t0.00022637\t0.00022434\t0.00022241\t0.0002204\t0.00021849\t0.0002165\t0.00021461\t0.00021264\t0.00021077\t0.00020882\t0.00020697\t0.00020504\t0.00020321\t0.0002013\t0.00019949\t0.00019761\t0.00019582\t0.00019395\t0.00019218\t0.00019034\t0.00018859\t0.00018676\t0.00018504\t0.00018323\t0.00018153\t0.00017974\t0.00017805\t0.00017628\t0.00017462\t0.00017287\t0.00017123\t0.0001695\t0.00016788\t0.00016617\t0.00016457\t0.00016288\t0.0001613\t0.00015963\t0.00015807\t0.00015642\t0.00015488\t0.00015325\t0.00015173\t0.00015012\t0.00014863\t0.00014703\t0.00014556\t0.00014398\t0.00014253\t0.00014097\t0.00013954\t0.000138\t0.00013659\t0.00013507\t0.00013368\t0.00013218\t0.00013081\t0.00012933\t0.00012798\t0.00012652\t0.00012519\t0.00012374\t0.00012243\t0.00012101\t0.00011972\t0.00011832\t0.00011704\t0.00011566\t0.0001144\t0.00011304\t0.00011181\t0.00011046\t0.00010925\t0.00010792\t0.00010673\t0.00010542\t0.00010425\t0.00010296\t0.00010181\t0.00010053\t9.94E-05\t9.81E-05\t9.70E-05\t9.58E-05\t9.47E-05\t9.35E-05\t9.24E-05\t9.12E-05\t9.01E-05\t8.90E-05\t8.79E-05\t8.68E-05\t8.57E-05\t8.46E-05\t8.36E-05\t8.25E-05\t8.15E-05\t8.04E-05\t7.94E-05\t7.83E-05\t7.73E-05\t7.63E-05\t7.53E-05\t7.43E-05\t7.34E-05\t7.23E-05\t7.14E-05\t7.04E-05\t6.95E-05\t6.85E-05\t6.76E-05\t6.66E-05\t6.58E-05\t6.48E-05\t6.40E-05\t6.30E-05\t6.22E-05\t6.13E-05\t6.05E-05\t5.95E-05\t5.88E-05\t5.78E-05\t5.71E-05\t5.62E-05\t5.54E-05\t5.45E-05\t5.38E-05\t5.30E-05\t5.22E-05\t5.14E-05\t5.07E-05\t4.99E-05\t4.92E-05\t4.84E-05\t4.77E-05\t4.69E-05\t4.62E-05\t4.55E-05\t4.48E-05\t4.40E-05\t4.34E-05\t4.27E-05\t4.20E-05\t4.13E-05\t4.07E-05\t4.00E-05\t3.94E-05\t3.87E-05\t3.81E-05\t3.74E-05\t3.69E-05\t3.62E-05\t3.56E-05\t3.49E-05\t3.44E-05\t3.37E-05\t3.32E-05\t3.26E-05\t3.21E-05\t3.15E-05\t3.10E-05\t3.03E-05\t2.99E-05\t2.93E-05\t2.88E-05\t2.82E-05\t2.78E-05\t2.72E-05\t2.67E-05\t2.61E-05\t2.57E-05\t2.52E-05\t2.48E-05\t2.42E-05\t2.39E-05\t2.33E-05\t2.29E-05\t2.24E-05\t2.20E-05\t2.15E-05\t2.11E-05\t2.06E-05\t2.02E-05\t1.99E-05\t1.93E-05\t1.88E-05\t1.87E-05\t1.82E-05\t1.79E-05\t1.74E-05\t1.71E-05\t1.66E-05\t1.63E-05\t1.58E-05\t1.56E-05\t1.51E-05\t1.49E-05\t1.45E-05\t1.42E-05\t1.38E-05\t1.36E-05\t1.32E-05\t1.30E-05\t0.00025758]"
  "Discrete-Time Integrator " : DiscreteIntegrator  gainval=100.0  ExternalReset=rising  SampleTime=-1  ICPrevOutput=DiscIntNeverNeededParam  ICPrevScaledInput=DiscIntNeverNeededParam
  "Gain " : Gain  Gain=6E-8
  Gain 1 : Gain  Gain=6E-8
  "Gain2 " : Gain  Gain=2e12
  NOT : Logic  Operator=NOT  IconShape=distinctive  AllPortsSameDT=off  OutDataTypeStr=boolean
  Offset1 : Constant  Value=0
  Offset2 : Constant  Value=0
  Product : Product
  Product1 : Product
  Quantizer : Quantizer  QuantizationInterval=1/Fs
  Quantizer1 : Quantizer  QuantizationInterval=1/Fs
  Quantizer2 : Quantizer  QuantizationInterval=1/Fs
  Sine Wave : Sin  Frequency=2*pi*500  SampleTime=1/Fs
  Zero-Order Hold : ZeroOrderHold  SampleTime=-1
  Zero-Order Hold1 : ZeroOrderHold  SampleTime=-1
  Zero-Order Hold2 : ZeroOrderHold  SampleTime=-1
  unit : Constant  SampleTime=-1
  Output : Outport
  wires:
  Product/1 -> "Discrete FIR Filter "/1
  Product1/1 -> "Discrete FIR Filter1 "/1
  "Discrete FIR Filter "/1 -> Abs/1
  "Discrete FIR Filter1 "/1 -> Abs1/1
  Abs1/1 -> Gain 1/1
  Abs/1 -> "Gain "/1
  "Gain "/1 -> Add/1
  Gain 1/1 -> Add/2
  Add/1 -> "Gain2 "/1
  "Gain2 "/1 -> "Discrete-Time Integrator "/1
  NOT/1 -> "D Flip-Flop "/3, "Discrete-Time Integrator "/2
  "Discrete-Time Integrator "/1 -> Compare To Constant/1
  Compare To Constant/1 -> "D Flip-Flop "/2
  "D Flip-Flop "/1 -> Delay/1
  unit/1 -> Cast To Boolean/1
  Cast To Boolean/1 -> "D Flip-Flop "/1
  Delay/1 -> NOT/1, Output/1
  Quantizer/1 -> Zero-Order Hold/1
  Zero-Order Hold/1 -> Product/1
  Zero-Order Hold1/1 -> Product1/2
  Quantizer1/1 -> Zero-Order Hold1/1
  Offset2/1 -> Add1/2
  Sine Wave/1 -> Add1/1
  Add1/1 -> Quantizer1/1
  Add2/1 -> Quantizer/1
  Cos Wave/1 -> Add2/2
  Offset1/1 -> Add2/1
  Quantizer2/1 -> Zero-Order Hold2/1
  In1/1 -> Quantizer2/1
  Zero-Order Hold2/1 -> Product1/1, Product/2
